simulink model "power_mosfet_device"  (R2025b)
settings: Solver=ode23tb  StartTime=0.0  StopTime=simlength  MaxStep=tc  RelTol=1e-3
values from neighbouring files (symbols this model uses):
  freq = 20e3    (= 20000)    [init_model.m]
  m = 0.5    [init_model.m]
  Rgate_turn_off = 1e-3    (= 0.001)    [init_model.m]
  Rgate_turn_on = 1    [init_model.m]
undefined symbols (not defined in the file or in its folder): cp_al, DThs_init, mosfet, Rth_mosfet_HA, Tambient, weigth
libraries: fl_lib x68, nesl_utility x32, simulink x4, advanced_mosfet_lib x2, basic_mosfet_lib x1, ee_lib x1
(part 1 of 2)
settings Model: SimulationMode=accelerator  Creator=dbagn  LastModifiedBy=dbagn

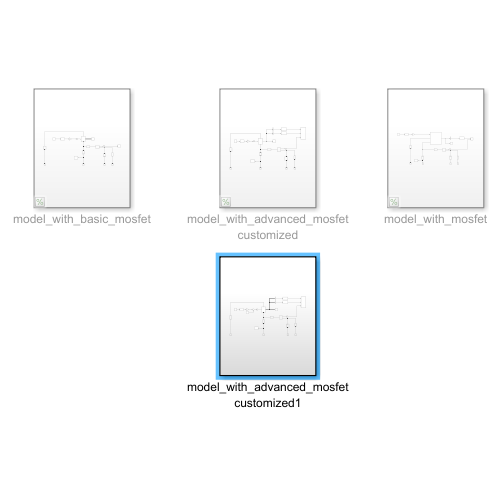
[thumbnail: Simulink's stored preview of the top-level diagram]
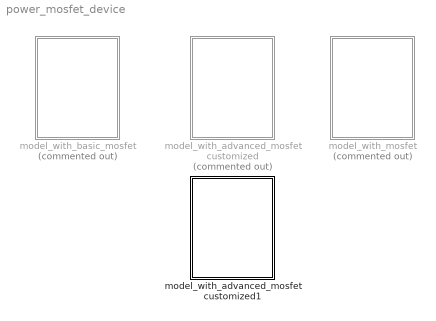
== system power_mosfet_device ==
  model_with_advanced_mosfet customized : Subsystem  Commented=on
  model_with_advanced_mosfet customized1 : Subsystem
  model_with_basic_mosfet : Subsystem  Commented=on
  model_with_mosfet : Subsystem  Commented=on

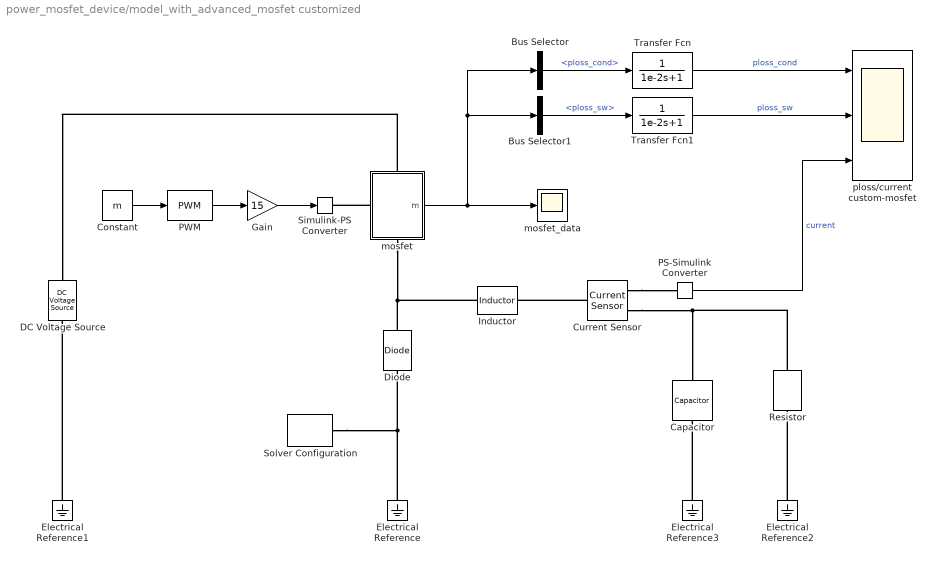
== system power_mosfet_device/model_with_advanced_mosfet customized ==
  Bus Selector : BusSelector  OutputSignals=basic_mosfet.ploss_cond
  Bus Selector1 : BusSelector  OutputSignals=basic_mosfet.ploss_sw
  Capacitor : fl_lib/Electrical/Electrical Elements/Capacitor  c=C F  r=1e-6 Ohm  g=0 1/Ohm  i_specify=off  i_priority=None  i=0 A  i_nominal_specify=off  i_nominal_value=1  i_nominal_unit=A  v_specify=off  v_priority=None  v=0 V  v_nominal_specify=off  v_nominal_value=1  v_nominal_unit=V  vc_specify=off  vc_priority=High  vc=0 V  vc_nominal_specify=off  vc_nominal_value=1  vc_nominal_unit=V
  Constant : Constant  Value=m
  Current Sensor : fl_lib/Electrical/Electrical Sensors/Current Sensor
  DC Voltage Source : fl_lib/Electrical/Electrical Sources/DC Voltage Source  v0=600 V
  Diode : fl_lib/Electrical/Electrical Elements/Diode  Vf=0.35 V  Ron=1e-3 Ohm  Goff=1e-8 1/Ohm  i_specify=off  i_priority=None  i=0 A  i_nominal_specify=off  i_nominal_value=1  i_nominal_unit=A  v_specify=off  v_priority=None  v=0 V  v_nominal_specify=off  v_nominal_value=1  v_nominal_unit=V
  Electrical Reference{,1..3} (4 alike) : fl_lib/Electrical/Electrical Elements/Electrical Reference
  Gain : Gain  Gain=15
  Inductor : fl_lib/Electrical/Electrical Elements/Inductor  l=L H  r=2e-3 Ohm  g=1e-9 1/Ohm  i_specify=off  i_priority=None  i=0 A  i_nominal_specify=off  i_nominal_value=1  i_nominal_unit=A  v_specify=off  v_priority=None  v=0 V  v_nominal_specify=off  v_nominal_value=1  v_nominal_unit=V  i_L_specify=off  i_L_priority=High  i_L=0 A  i_L_nominal_specify=off  i_L_nominal_value=1  i_L_nominal_unit=A
  PS-Simulink Converter : nesl_utility/PS-Simulink Converter  PhysicalDomain=network_engine_domain  SubClassName=ps_output  LeftPortType=input  RightPortType=output  PseudoPeriodic=off  Frequencies=[]  VectorFormat=1-D array  Unit=A  AffineConversion=off
  PWM : simulink/Discontinuities/PWM  DisableCoverage=on  Period=1/freq  InitialDelay=0  DisallowZeroDutyCycle=off  RunAtFixedTimeIntervals=off  SampleTime=0.1
  Resistor : fl_lib/Electrical/Electrical Elements/Resistor  R=300/200 Ohm  i_specify=off  i_priority=None  i=0 A  i_nominal_specify=off  i_nominal_value=1  i_nominal_unit=A  v_specify=off  v_priority=None  v=0 V  v_nominal_specify=off  v_nominal_value=1  v_nominal_unit=V
  Simulink-PS Converter : nesl_utility/Simulink-PS Converter  PhysicalDomain=network_engine_domain  SubClassName=ps_input  LeftPortType=input  RightPortType=output  PseudoPeriodic=off  Frequencies=[]  NoiseDistribution=none  NoiseParameters=[]  Unit=1  AffineConversion=off  FilteringAndDerivatives=provide  SimscapeFilterOrder=1  InputFilterTimeConstant=0.001  UdotUserProvided=0
  Solver Configuration : nesl_utility/Solver Configuration  PhysicalDomain=network_engine_domain  SubClassName=solver  LeftPortType=input  RightPortType=generic  Tones=[]  Harmonics=[]  SimulateNoise=off  Profile=off  UseLocalSampling=off  EnableSwitchedLinearOptims=on  FrequencyDomain=off  UseCCode=off  RelTol=0.001  AbsTol=0.001  MinStep=1e-09  ToWorkspace=off  RevertToSquareIcSolve=off  NumHomotopyIterations=100  PhasorMode=off  PhasorModeNumHarmonics=1  ConsistencySolver=NEWTON_XTOL_AFTER_FTOL  IndexReductionMethod=DerivativeReplacement  DoDC=on  ResidualTolerance=1e-09  ConsistencyTolSource=GLOBAL  ConsistencyAbsTol=0.001  ConsistencyRelTol=0.001  ConsistencyTolFactor=0.001  UseLocalSolver=on  LocalSolverChoice=NE_BACKWARD_EULER_ADVANCER  ResolveIndetEquations=on  FunctionEvalNumThread=1  LocalSolverSampleTime=tc  DoFixedCost=on  MaxNonlinIter=3  MaxModeIter=2  ComputeImpulses=off  ImpulseIterations=2  LinearAlgebra=auto  LinearAlgebraNumThread=0  EquationFormulation=NE_TIME_EF  DelaysMemoryBudget=1024  AutomaticFiltering=on  FilteringTimeConstant=0.001  PartitionStorageMethod=AS_NEEDED  PartitionMemoryBudget=1024  PartitionMethod=ROBUST  MultibodyUseLocalSolver=off  MultibodyLocalSolverChoice=ODE1  MultibodyLocalSolverSampleTime=0.001
  Transfer Fcn : TransferFcn  Denominator=[1e-2 1]
  Transfer Fcn1 : TransferFcn  Denominator=[1e-2 1]
  mosfet : Subsystem  mask{Rds_on_m=mosfet.inv.Rds_on, Vth_m=mosfet.inv.Vth, Vdon_diode_m=mosfet.inv.Vdon_diode, Rdon_diode_m=mosfet.inv.Rdon_diode, g_fs_m=mosfet.inv.g_fs, Cgs_m=mosfet.inv.Cgs, Cgd_m=mosfet.inv.Cgd, Cds_m=mosfet.inv.Cds, Eon_m=mosfet.inv.Eon, Eoff_m=mosfet.inv.Eoff, Err_m=mosfet.inv.Erec, Voff_sw_loss_m=mosfet.inv.Voff_sw_losses, Ion_sw_loss_m=mosfet.inv.Ion_sw_losses, Rgate_internal_m=mosfet.inv.Rgate_internal, Rgate_turn_on_m=Rgate_turn_on, Rgate_turn_off_m=Rgate_turn_off, Lstray_m=mosfet.inv.Lstray_module}
      mask prompts: Rds_on_m "Rds_on (Ohm)"; Vth_m "Vth (V)"; Vdon_diode_m "Vdon_diode (V)"; Rdon_diode_m "Rdon_diode (Ohm)"; g_fs_m "g_fs (A/V)"; Cgs_m "Cgs (F)"; Cgd_m "Cgd (F)"; Cds_m "Cds (F)"; Eon_m "Eon (J)"; Eoff_m "Eoff (J)"; Err_m "Err (J)"; Voff_sw_loss_m "Voff_sw_loss (V)"; Ion_sw_loss_m "Ion _sw_loss (A)"; Rgate_internal_m "Rgate internal (Ohm)"; Rgate_turn_on_m "Rgate turn on (Ohm)"; Rgate_turn_off_m "Rgate turn off (Ohm)"; Lstray_m "Lstray module (H)"
      settings: PortSchema="{\"entries\":[{\"content\":{\"sides\":[{\"content\":{\"connectorIds\":[\"LConn1\"]},\"type\":\"ConnectorPlacement.EquallySpacedRectSide\",\"uuid\":\"325dc963-858c-47f0-8995-f323ab4d9c46\"},{\"content\":{\"connectorIds\":[\"Out1\"],\"side\":\"RIGHT\"},\"type\":\"ConnectorPlacement.EquallySpacedRectSide\",\"uuid\":\"e9e66084-ecb2-40fb-9a1e-77677e0cc1df\"},{\"content\":{\"connectorIds\":[\"LConn2\"],\"side\":\"TOP\"},\"type\":\"ConnectorPlacement.EquallySpacedRectSide\",\"uuid\":\"9480d797-f2f6-459b-bb7c-d63861b57fde\"},{\"content\":{\"connectorIds\":[\"RConn1\"],\"side\":\"BOTTOM\"},\"type\":\"ConnectorPlacement.EquallySpacedRectSide\",\"uuid\":\"b13176d9-73b9-4822-9a0d-ec75065272bc\"}]},\"type\":\"ConnectorPlacement.EquallySpacedConnector\",\"uuid\":\"5e4a07d9-f5e8-4613-9049-5a866b5d2453\"}],\"packageUris\":[\"http://schema.mathworks.com/mf0/Connector/R2020b\"],\"version\":\"1.0\"}"
  mosfet_data : Scope
      settings: SampleTime=tc  ActiveDisplayYMinimum=-130.18028660470713  ActiveDisplayYMaximum=1171.6225788682864
  ploss/current custom-mosfet : Scope  NumInputPorts=3
      settings: ActiveDisplayYMinimum=-4.6879645806866894E+6  ActiveDisplayYMaximum=4.2191681226180211E+7
  wires:
  Gain/1 -> Simulink-PS Converter/1
  mosfet/1(m) -> Bus Selector1/1, Bus Selector/1, mosfet_data/1
  Constant/1 -> PWM/1
  PWM/1 -> Gain/1
  Bus Selector/1 -> Transfer Fcn/1  "<ploss_cond>"
  Transfer Fcn/1 -> ploss/current custom-mosfet/1  "ploss_cond"
  PS-Simulink Converter/1 -> ploss/current custom-mosfet/3  "current"
  Bus Selector1/1 -> Transfer Fcn1/1  "<ploss_sw>"
  Transfer Fcn1/1 -> ploss/current custom-mosfet/2  "ploss_sw"
  connections:
  Electrical Reference1/LConn1 -- DC Voltage Source/RConn1
  mosfet/LConn1 -- Simulink-PS Converter/RConn1
  mosfet/LConn2 -- Diode/RConn1 -- Inductor/LConn1
  Resistor/LConn1 -- Capacitor/LConn1 -- Current Sensor/RConn2
  Electrical Reference2/LConn1 -- Resistor/RConn1
  Electrical Reference3/LConn1 -- Capacitor/RConn1
  Solver Configuration/RConn1 -- Electrical Reference/LConn1 -- Diode/LConn1
  mosfet/RConn1 -- DC Voltage Source/LConn1
  Current Sensor/LConn1 -- Inductor/RConn1
  Current Sensor/RConn1 -- PS-Simulink Converter/LConn1

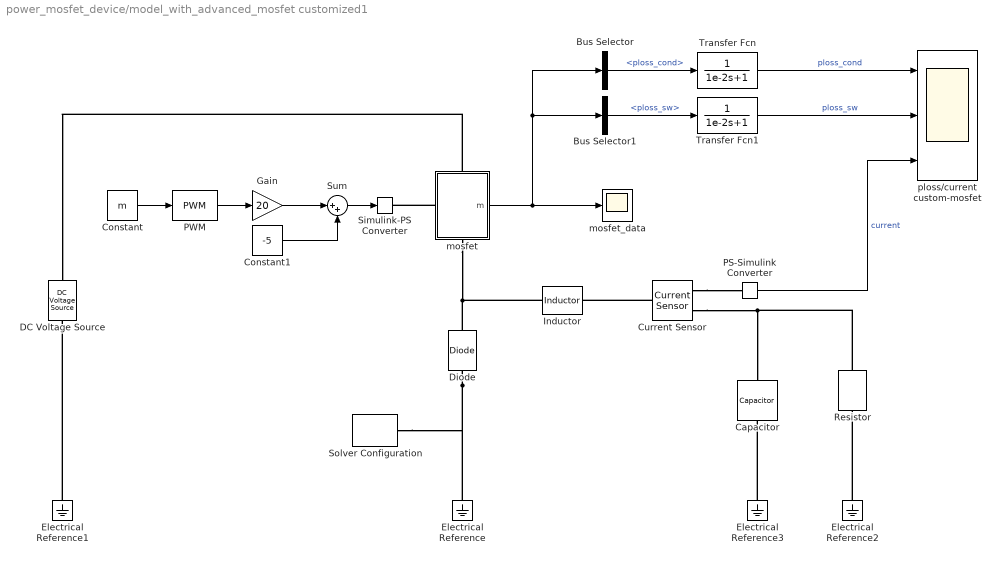
== system power_mosfet_device/model_with_advanced_mosfet customized1 ==
  Bus Selector : BusSelector  OutputSignals=basic_mosfet.ploss_cond
  Bus Selector1 : BusSelector  OutputSignals=basic_mosfet.ploss_sw
  Capacitor : fl_lib/Electrical/Electrical Elements/Capacitor  c=C F  r=1e-6 Ohm  g=0 1/Ohm  i_specify=off  i_priority=None  i=0 A  i_nominal_specify=off  i_nominal_value=1  i_nominal_unit=A  v_specify=off  v_priority=None  v=0 V  v_nominal_specify=off  v_nominal_value=1  v_nominal_unit=V  vc_specify=off  vc_priority=High  vc=0 V  vc_nominal_specify=off  vc_nominal_value=1  vc_nominal_unit=V
  Constant : Constant  Value=m
  Constant1 : Constant  Value=-5
  Current Sensor : fl_lib/Electrical/Electrical Sensors/Current Sensor
  DC Voltage Source : fl_lib/Electrical/Electrical Sources/DC Voltage Source  v0=600 V
  Diode : fl_lib/Electrical/Electrical Elements/Diode  Vf=0.35 V  Ron=1e-3 Ohm  Goff=1e-8 1/Ohm  i_specify=off  i_priority=None  i=0 A  i_nominal_specify=off  i_nominal_value=1  i_nominal_unit=A  v_specify=off  v_priority=None  v=0 V  v_nominal_specify=off  v_nominal_value=1  v_nominal_unit=V
  Electrical Reference{,1..3} (4 alike) : fl_lib/Electrical/Electrical Elements/Electrical Reference
  Gain : Gain  Gain=20
  Inductor : fl_lib/Electrical/Electrical Elements/Inductor  l=L H  r=2e-3 Ohm  g=1e-9 1/Ohm  i_specify=off  i_priority=None  i=0 A  i_nominal_specify=off  i_nominal_value=1  i_nominal_unit=A  v_specify=off  v_priority=None  v=0 V  v_nominal_specify=off  v_nominal_value=1  v_nominal_unit=V  i_L_specify=off  i_L_priority=High  i_L=0 A  i_L_nominal_specify=off  i_L_nominal_value=1  i_L_nominal_unit=A
  PS-Simulink Converter : nesl_utility/PS-Simulink Converter  PhysicalDomain=network_engine_domain  SubClassName=ps_output  LeftPortType=input  RightPortType=output  PseudoPeriodic=off  Frequencies=[]  VectorFormat=1-D array  Unit=A  AffineConversion=off
  PWM : simulink/Discontinuities/PWM  DisableCoverage=on  Period=1/freq  InitialDelay=0  DisallowZeroDutyCycle=off  RunAtFixedTimeIntervals=off  SampleTime=0.1
  Resistor : fl_lib/Electrical/Electrical Elements/Resistor  R=300/200 Ohm  i_specify=off  i_priority=None  i=0 A  i_nominal_specify=off  i_nominal_value=1  i_nominal_unit=A  v_specify=off  v_priority=None  v=0 V  v_nominal_specify=off  v_nominal_value=1  v_nominal_unit=V
  Simulink-PS Converter : nesl_utility/Simulink-PS Converter  PhysicalDomain=network_engine_domain  SubClassName=ps_input  LeftPortType=input  RightPortType=output  PseudoPeriodic=off  Frequencies=[]  NoiseDistribution=none  NoiseParameters=[]  Unit=1  AffineConversion=off  FilteringAndDerivatives=provide  SimscapeFilterOrder=1  InputFilterTimeConstant=0.001  UdotUserProvided=0
  Solver Configuration : nesl_utility/Solver Configuration  PhysicalDomain=network_engine_domain  SubClassName=solver  LeftPortType=input  RightPortType=generic  Tones=[]  Harmonics=[]  SimulateNoise=off  Profile=off  UseLocalSampling=off  EnableSwitchedLinearOptims=on  FrequencyDomain=off  UseCCode=off  RelTol=0.001  AbsTol=0.001  MinStep=1e-09  ToWorkspace=off  RevertToSquareIcSolve=off  NumHomotopyIterations=100  PhasorMode=off  PhasorModeNumHarmonics=1  ConsistencySolver=NEWTON_XTOL_AFTER_FTOL  IndexReductionMethod=DerivativeReplacement  DoDC=on  ResidualTolerance=1e-09  ConsistencyTolSource=GLOBAL  ConsistencyAbsTol=0.001  ConsistencyRelTol=0.001  ConsistencyTolFactor=0.001  UseLocalSolver=on  LocalSolverChoice=NE_BACKWARD_EULER_ADVANCER  ResolveIndetEquations=on  FunctionEvalNumThread=1  LocalSolverSampleTime=tc  DoFixedCost=on  MaxNonlinIter=3  MaxModeIter=2  ComputeImpulses=off  ImpulseIterations=2  LinearAlgebra=auto  LinearAlgebraNumThread=0  EquationFormulation=NE_TIME_EF  DelaysMemoryBudget=1024  AutomaticFiltering=on  FilteringTimeConstant=0.001  PartitionStorageMethod=AS_NEEDED  PartitionMemoryBudget=1024  PartitionMethod=ROBUST  MultibodyUseLocalSolver=off  MultibodyLocalSolverChoice=ODE1  MultibodyLocalSolverSampleTime=0.001
  Sum : Sum  Inputs=|++
  Transfer Fcn : TransferFcn  Denominator=[1e-2 1]
  Transfer Fcn1 : TransferFcn  Denominator=[1e-2 1]
  mosfet : Subsystem  mask{Rds_on_m=mosfet.inv.Rds_on, Vth_m=mosfet.inv.Vth, Vdon_diode_m=mosfet.inv.Vdon_diode, Rdon_diode_m=mosfet.inv.Rdon_diode, g_fs_m=mosfet.inv.g_fs, Cgs_m=mosfet.inv.Cgs, Cgd_m=mosfet.inv.Cgd, Cds_m=mosfet.inv.Cds, Eon_m=mosfet.inv.Eon, Eoff_m=mosfet.inv.Eoff, Err_m=mosfet.inv.Erec, Voff_sw_loss_m=mosfet.inv.Voff_sw_losses, Ion_sw_loss_m=mosfet.inv.Ion_sw_losses, Rgate_internal_m=mosfet.inv.Rgate_internal, Rgate_turn_on_m=Rgate_turn_on, Rgate_turn_off_m=Rgate_turn_off, Lstray_m=mosfet.inv.Lstray_module}
      mask prompts: Rds_on_m "Rds_on (Ohm)"; Vth_m "Vth (V)"; Vdon_diode_m "Vdon_diode (V)"; Rdon_diode_m "Rdon_diode (Ohm)"; g_fs_m "g_fs (A/V)"; Cgs_m "Cgs (F)"; Cgd_m "Cgd (F)"; Cds_m "Cds (F)"; Eon_m "Eon (J)"; Eoff_m "Eoff (J)"; Err_m "Err (J)"; Voff_sw_loss_m "Voff_sw_loss (V)"; Ion_sw_loss_m "Ion _sw_loss (A)"; Rgate_internal_m "Rgate internal (Ohm)"; Rgate_turn_on_m "Rgate turn on (Ohm)"; Rgate_turn_off_m "Rgate turn off (Ohm)"; Lstray_m "Lstray module (H)"
      settings: PortSchema="{\"entries\":[{\"content\":{\"sides\":[{\"content\":{\"connectorIds\":[\"LConn1\"]},\"type\":\"ConnectorPlacement.EquallySpacedRectSide\",\"uuid\":\"325dc963-858c-47f0-8995-f323ab4d9c46\"},{\"content\":{\"connectorIds\":[\"Out1\"],\"side\":\"RIGHT\"},\"type\":\"ConnectorPlacement.EquallySpacedRectSide\",\"uuid\":\"e9e66084-ecb2-40fb-9a1e-77677e0cc1df\"},{\"content\":{\"connectorIds\":[\"LConn2\"],\"side\":\"TOP\"},\"type\":\"ConnectorPlacement.EquallySpacedRectSide\",\"uuid\":\"9480d797-f2f6-459b-bb7c-d63861b57fde\"},{\"content\":{\"connectorIds\":[\"RConn1\"],\"side\":\"BOTTOM\"},\"type\":\"ConnectorPlacement.EquallySpacedRectSide\",\"uuid\":\"b13176d9-73b9-4822-9a0d-ec75065272bc\"}]},\"type\":\"ConnectorPlacement.EquallySpacedConnector\",\"uuid\":\"5e4a07d9-f5e8-4613-9049-5a866b5d2453\"}],\"packageUris\":[\"http://schema.mathworks.com/mf0/Connector/R2020b\"],\"version\":\"1.0\"}"
  mosfet_data : Scope
      settings: SampleTime=tc  ActiveDisplayYMinimum=-1205.322347971507  ActiveDisplayYMaximum=2898.4652473437918
  ploss/current custom-mosfet : Scope  NumInputPorts=3
      settings: ActiveDisplayYMinimum=-1.5081366929735125  ActiveDisplayYMaximum=13.573230236761617
  wires:
  Transfer Fcn1/1 -> ploss/current custom-mosfet/2  "ploss_sw"
  Bus Selector1/1 -> Transfer Fcn1/1  "<ploss_sw>"
  PS-Simulink Converter/1 -> ploss/current custom-mosfet/3  "current"
  Transfer Fcn/1 -> ploss/current custom-mosfet/1  "ploss_cond"
  Bus Selector/1 -> Transfer Fcn/1  "<ploss_cond>"
  PWM/1 -> Gain/1
  Constant/1 -> PWM/1
  mosfet/1(m) -> mosfet_data/1, Bus Selector/1, Bus Selector1/1
  Gain/1 -> Sum/1
  Sum/1 -> Simulink-PS Converter/1
  Constant1/1 -> Sum/2
  connections:
  Current Sensor/RConn1 -- PS-Simulink Converter/LConn1
  Current Sensor/LConn1 -- Inductor/RConn1
  mosfet/RConn1 -- DC Voltage Source/LConn1
  Diode/LConn1 -- Electrical Reference/LConn1 -- Solver Configuration/RConn1
  Electrical Reference3/LConn1 -- Capacitor/RConn1
  Electrical Reference2/LConn1 -- Resistor/RConn1
  Current Sensor/RConn2 -- Capacitor/LConn1 -- Resistor/LConn1
  Inductor/LConn1 -- Diode/RConn1 -- mosfet/LConn2
  mosfet/LConn1 -- Simulink-PS Converter/RConn1
  Electrical Reference1/LConn1 -- DC Voltage Source/RConn1

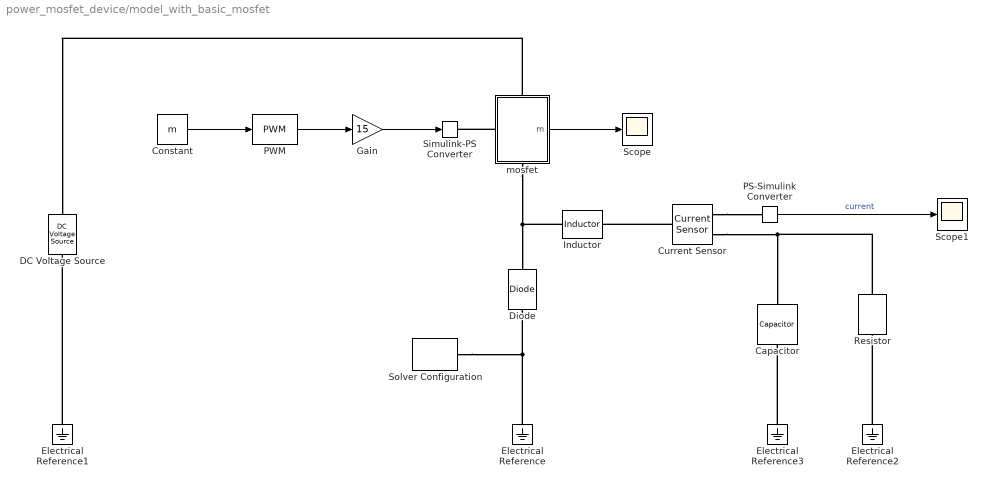
== system power_mosfet_device/model_with_basic_mosfet ==
  Capacitor : fl_lib/Electrical/Electrical Elements/Capacitor  c=C F  r=1e-6 Ohm  g=0 1/Ohm  i_specify=off  i_priority=None  i=0 A  i_nominal_specify=off  i_nominal_value=1  i_nominal_unit=A  v_specify=off  v_priority=None  v=0 V  v_nominal_specify=off  v_nominal_value=1  v_nominal_unit=V  vc_specify=off  vc_priority=High  vc=0 V  vc_nominal_specify=off  vc_nominal_value=1  vc_nominal_unit=V
  Constant : Constant  Value=m
  Current Sensor : fl_lib/Electrical/Electrical Sensors/Current Sensor
  DC Voltage Source : fl_lib/Electrical/Electrical Sources/DC Voltage Source  v0=600 V
  Diode : fl_lib/Electrical/Electrical Elements/Diode  Vf=0.35 V  Ron=1e-3 Ohm  Goff=1e-8 1/Ohm  i_specify=off  i_priority=None  i=0 A  i_nominal_specify=off  i_nominal_value=1  i_nominal_unit=A  v_specify=off  v_priority=None  v=0 V  v_nominal_specify=off  v_nominal_value=1  v_nominal_unit=V
  Electrical Reference{,1..3} (4 alike) : fl_lib/Electrical/Electrical Elements/Electrical Reference
  Gain : Gain  Gain=15
  Inductor : fl_lib/Electrical/Electrical Elements/Inductor  l=L H  r=2e-3 Ohm  g=1e-9 1/Ohm  i_specify=off  i_priority=None  i=0 A  i_nominal_specify=off  i_nominal_value=1  i_nominal_unit=A  v_specify=off  v_priority=None  v=0 V  v_nominal_specify=off  v_nominal_value=1  v_nominal_unit=V  i_L_specify=off  i_L_priority=High  i_L=0 A  i_L_nominal_specify=off  i_L_nominal_value=1  i_L_nominal_unit=A
  PS-Simulink Converter : nesl_utility/PS-Simulink Converter  PhysicalDomain=network_engine_domain  SubClassName=ps_output  LeftPortType=input  RightPortType=output  PseudoPeriodic=off  Frequencies=[]  VectorFormat=1-D array  Unit=A  AffineConversion=off
  PWM : simulink/Discontinuities/PWM  DisableCoverage=on  Period=1/freq  InitialDelay=0  DisallowZeroDutyCycle=off  RunAtFixedTimeIntervals=off  SampleTime=0.1
  Resistor : fl_lib/Electrical/Electrical Elements/Resistor  R=300/200 Ohm  i_specify=off  i_priority=None  i=0 A  i_nominal_specify=off  i_nominal_value=1  i_nominal_unit=A  v_specify=off  v_priority=None  v=0 V  v_nominal_specify=off  v_nominal_value=1  v_nominal_unit=V
  Scope : Scope
      settings: SampleTime=tc  ActiveDisplayYMinimum=-75.266839616145688  ActiveDisplayYMaximum=677.40155654531134
  Scope1 : Scope
      settings: SampleTime=tc  ActiveDisplayYMinimum=159.93430922640852  ActiveDisplayYMaximum=242.39946565162148  DataLoggingVariableName=ScopeData2
  Simulink-PS Converter : nesl_utility/Simulink-PS Converter  PhysicalDomain=network_engine_domain  SubClassName=ps_input  LeftPortType=input  RightPortType=output  PseudoPeriodic=off  Frequencies=[]  NoiseDistribution=none  NoiseParameters=[]  Unit=1  AffineConversion=off  FilteringAndDerivatives=provide  SimscapeFilterOrder=1  InputFilterTimeConstant=0.001  UdotUserProvided=0
  Solver Configuration : nesl_utility/Solver Configuration  PhysicalDomain=network_engine_domain  SubClassName=solver  LeftPortType=input  RightPortType=generic  Tones=[]  Harmonics=[]  SimulateNoise=off  Profile=off  UseLocalSampling=off  EnableSwitchedLinearOptims=on  FrequencyDomain=off  UseCCode=off  RelTol=0.001  AbsTol=0.001  MinStep=1e-09  ToWorkspace=off  RevertToSquareIcSolve=off  NumHomotopyIterations=100  PhasorMode=off  PhasorModeNumHarmonics=1  ConsistencySolver=NEWTON_XTOL_AFTER_FTOL  IndexReductionMethod=DerivativeReplacement  DoDC=on  ResidualTolerance=1e-09  ConsistencyTolSource=GLOBAL  ConsistencyAbsTol=0.001  ConsistencyRelTol=0.001  ConsistencyTolFactor=0.001  UseLocalSolver=on  LocalSolverChoice=NE_BACKWARD_EULER_ADVANCER  ResolveIndetEquations=on  FunctionEvalNumThread=1  LocalSolverSampleTime=tc  DoFixedCost=on  MaxNonlinIter=3  MaxModeIter=2  ComputeImpulses=off  ImpulseIterations=2  LinearAlgebra=auto  LinearAlgebraNumThread=0  EquationFormulation=NE_TIME_EF  DelaysMemoryBudget=1024  AutomaticFiltering=on  FilteringTimeConstant=0.001  PartitionStorageMethod=AS_NEEDED  PartitionMemoryBudget=1024  PartitionMethod=ROBUST  MultibodyUseLocalSolver=off  MultibodyLocalSolverChoice=ODE1  MultibodyLocalSolverSampleTime=0.001
  mosfet : Subsystem  mask{Rds_on=mosfet.inv.Rds_on, Vth=mosfet.inv.Vth, Csnubber=mosfet.inv.Csnubber, Rsnubber=mosfet.inv.Rsnubber, Lstray=mosfet.inv.Lstray_module/2, Vdon_diode=mosfet.inv.Vdon_diode, Rdon_diode=mosfet.inv.Rdon_diode, g_fs=mosfet.inv.g_fs}
      mask prompts: Rds_on "Rds_on (Ohm)"; Vth "Vth (V)"; Csnubber "Csnubber (F)"; Rsnubber "Rsnubber (Ohm)"; Lstray "Lstray (H)"; Vdon_diode "Vdon_diode (V)"; Rdon_diode "Rdon_diode (Ohm)"; g_fs "g_fs (A/V)"
      settings: PortSchema="{\"entries\":[{\"content\":{\"sides\":[{\"content\":{\"connectorIds\":[\"LConn1\"]},\"type\":\"ConnectorPlacement.EquallySpacedRectSide\",\"uuid\":\"325dc963-858c-47f0-8995-f323ab4d9c46\"},{\"content\":{\"connectorIds\":[\"Out1\"],\"side\":\"RIGHT\"},\"type\":\"ConnectorPlacement.EquallySpacedRectSide\",\"uuid\":\"e9e66084-ecb2-40fb-9a1e-77677e0cc1df\"},{\"content\":{\"connectorIds\":[\"LConn2\"],\"side\":\"TOP\"},\"type\":\"ConnectorPlacement.EquallySpacedRectSide\",\"uuid\":\"9480d797-f2f6-459b-bb7c-d63861b57fde\"},{\"content\":{\"connectorIds\":[\"RConn1\"],\"side\":\"BOTTOM\"},\"type\":\"ConnectorPlacement.EquallySpacedRectSide\",\"uuid\":\"b13176d9-73b9-4822-9a0d-ec75065272bc\"}]},\"type\":\"ConnectorPlacement.EquallySpacedConnector\",\"uuid\":\"5e4a07d9-f5e8-4613-9049-5a866b5d2453\"}],\"packageUris\":[\"http://schema.mathworks.com/mf0/Connector/R2020b\"],\"version\":\"1.0\"}"
  wires:
  PWM/1 -> Gain/1
  Constant/1 -> PWM/1
  mosfet/1(m) -> Scope/1
  Gain/1 -> Simulink-PS Converter/1
  PS-Simulink Converter/1 -> Scope1/1  "current"
  connections:
  mosfet/RConn1 -- DC Voltage Source/LConn1
  Electrical Reference/LConn1 -- Solver Configuration/RConn1 -- Diode/LConn1
  mosfet/LConn2 -- Inductor/LConn1 -- Diode/RConn1
  mosfet/LConn1 -- Simulink-PS Converter/RConn1
  Electrical Reference1/LConn1 -- DC Voltage Source/RConn1
  Current Sensor/RConn2 -- Resistor/LConn1 -- Capacitor/LConn1
  Current Sensor/LConn1 -- Inductor/RConn1
  Current Sensor/RConn1 -- PS-Simulink Converter/LConn1
  Electrical Reference2/LConn1 -- Resistor/RConn1
  Electrical Reference3/LConn1 -- Capacitor/RConn1

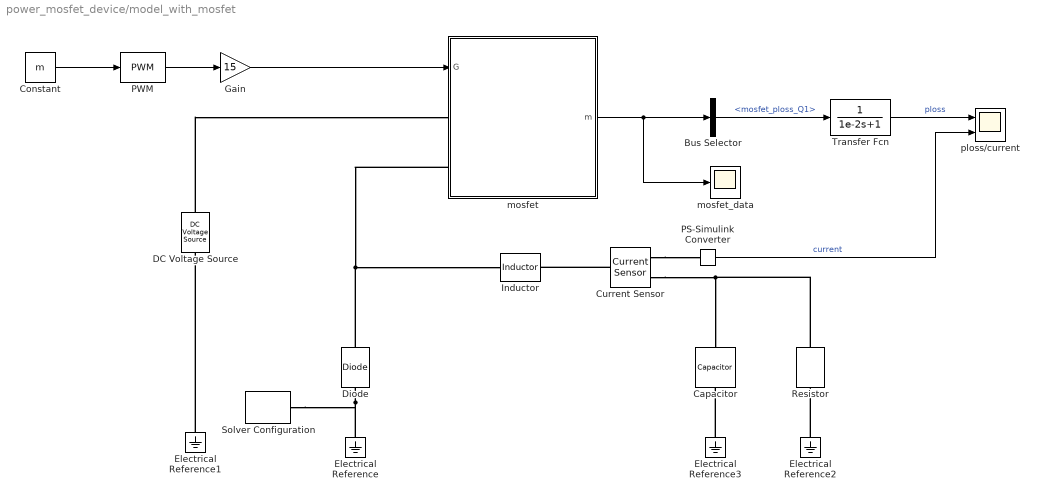
== system power_mosfet_device/model_with_mosfet ==
  Bus Selector : BusSelector  OutputSignals=mosfet_ploss_Q1
  Capacitor : fl_lib/Electrical/Electrical Elements/Capacitor  c=C F  r=1e-6 Ohm  g=0 1/Ohm  i_specify=off  i_priority=None  i=0 A  i_nominal_specify=off  i_nominal_value=1  i_nominal_unit=A  v_specify=off  v_priority=None  v=0 V  v_nominal_specify=off  v_nominal_value=1  v_nominal_unit=V  vc_specify=off  vc_priority=High  vc=0 V  vc_nominal_specify=off  vc_nominal_value=1  vc_nominal_unit=V
  Constant : Constant  Value=m
  Current Sensor : fl_lib/Electrical/Electrical Sensors/Current Sensor
  DC Voltage Source : fl_lib/Electrical/Electrical Sources/DC Voltage Source  v0=600 V
  Diode : fl_lib/Electrical/Electrical Elements/Diode  Vf=0.35 V  Ron=1e-3 Ohm  Goff=1e-8 1/Ohm  i_specify=off  i_priority=None  i=0 A  i_nominal_specify=off  i_nominal_value=1  i_nominal_unit=A  v_specify=off  v_priority=None  v=0 V  v_nominal_specify=off  v_nominal_value=1  v_nominal_unit=V
  Electrical Reference{,1..3} (4 alike) : fl_lib/Electrical/Electrical Elements/Electrical Reference
  Gain : Gain  Gain=15
  Inductor : fl_lib/Electrical/Electrical Elements/Inductor  l=L H  r=2e-3 Ohm  g=1e-9 1/Ohm  i_specify=off  i_priority=None  i=0 A  i_nominal_specify=off  i_nominal_value=1  i_nominal_unit=A  v_specify=off  v_priority=None  v=0 V  v_nominal_specify=off  v_nominal_value=1  v_nominal_unit=V  i_L_specify=off  i_L_priority=High  i_L=0 A  i_L_nominal_specify=off  i_L_nominal_value=1  i_L_nominal_unit=A
  PS-Simulink Converter : nesl_utility/PS-Simulink Converter  PhysicalDomain=network_engine_domain  SubClassName=ps_output  LeftPortType=input  RightPortType=output  PseudoPeriodic=off  Frequencies=[]  VectorFormat=1-D array  Unit=A  AffineConversion=off
  PWM : simulink/Discontinuities/PWM  DisableCoverage=on  Period=1/freq  InitialDelay=0  DisallowZeroDutyCycle=off  RunAtFixedTimeIntervals=off  SampleTime=0.1
  Resistor : fl_lib/Electrical/Electrical Elements/Resistor  R=300/200 Ohm  i_specify=off  i_priority=None  i=0 A  i_nominal_specify=off  i_nominal_value=1  i_nominal_unit=A  v_specify=off  v_priority=None  v=0 V  v_nominal_specify=off  v_nominal_value=1  v_nominal_unit=V
  Solver Configuration : nesl_utility/Solver Configuration  PhysicalDomain=network_engine_domain  SubClassName=solver  LeftPortType=input  RightPortType=generic  Tones=[]  Harmonics=[]  SimulateNoise=off  Profile=off  UseLocalSampling=off  EnableSwitchedLinearOptims=on  FrequencyDomain=off  UseCCode=off  RelTol=0.001  AbsTol=0.001  MinStep=1e-09  ToWorkspace=off  RevertToSquareIcSolve=off  NumHomotopyIterations=100  PhasorMode=off  PhasorModeNumHarmonics=1  ConsistencySolver=NEWTON_XTOL_AFTER_FTOL  IndexReductionMethod=DerivativeReplacement  DoDC=on  ResidualTolerance=1e-09  ConsistencyTolSource=GLOBAL  ConsistencyAbsTol=0.001  ConsistencyRelTol=0.001  ConsistencyTolFactor=0.001  UseLocalSolver=on  LocalSolverChoice=NE_BACKWARD_EULER_ADVANCER  ResolveIndetEquations=on  FunctionEvalNumThread=1  LocalSolverSampleTime=tc  DoFixedCost=on  MaxNonlinIter=3  MaxModeIter=2  ComputeImpulses=off  ImpulseIterations=2  LinearAlgebra=auto  LinearAlgebraNumThread=0  EquationFormulation=NE_TIME_EF  DelaysMemoryBudget=1024  AutomaticFiltering=on  FilteringTimeConstant=0.001  PartitionStorageMethod=AS_NEEDED  PartitionMemoryBudget=1024  PartitionMethod=ROBUST  MultibodyUseLocalSolver=off  MultibodyLocalSolverChoice=ODE1  MultibodyLocalSolverSampleTime=0.001
  Transfer Fcn : TransferFcn  Denominator=[1e-2 1]
  mosfet : Subsystem  mask{mass_heatsink=weigth, specific_heat=cp_al, rth_mosfet_HA=Rth_mosfet_HA, rth_mosfet_JH=mosfet.inv.Rth_switch_JH, Rds_on=mosfet.inv.Rds_on, Vth=mosfet.inv.Vth, Eon=mosfet.inv.Eon, Eoff=mosfet.inv.Eoff, Voff_sw_loss=mosfet.inv.Voff_sw_losses, Ion_sw_loss=mosfet.inv.Ion_sw_losses, Vdon_diode=mosfet.inv.Vdon_diode, Rdon_diode=mosfet.inv.Rdon_diode, JunctionTermalMass=mosfet.inv.JunctionTermalMass, Tambient=Tambient, DThs_init=DThs_init, Csnubber=mosfet.inv.Csnubber, Rsnubber=mosfet.inv.Rsnubber}
      mask prompts: mass_heatsink "Mass Heatsink (kg)"; specific_heat "Specific Heat (J/K/kg)"; rth_mosfet_HA "Thermal Resistance HA (K/W)"; rth_mosfet_JH "Thermal Resistance JH (K/W)"; Rds_on "Rds_on (Ohm)"; Vth "Vth (V)"; Eon "Eon (J)"; Eoff "Eoff (J)"; Voff_sw_loss "Voff_sw_loss (V)"; Ion_sw_loss "Ion_sw_loss (A)"; Vdon_diode "Vdon_diode (V)"; Rdon_diode "Rdon_diode (Ohm)"; JunctionTermalMass "JunctionTermalMass (J/K)"; Tambient "Tambient (degC)"; DThs_init "DThs_init (degC)"; Csnubber "Csnubber (F)"; Rsnubber "Rsnubber (Ohm)"
  mosfet_data : Scope
      settings: SampleTime=tc  ActiveDisplayYMinimum=-162.71512014835841  ActiveDisplayYMaximum=162.83727252978858
  ploss/current : Scope  NumInputPorts=2
      settings: ActiveDisplayYMinimum=112.87858768707648  ActiveDisplayYMaximum=429.36143412410507
  wires:
  PS-Simulink Converter/1 -> ploss/current/2  "current"
  Transfer Fcn/1 -> ploss/current/1  "ploss"
  Bus Selector/1 -> Transfer Fcn/1  "<mosfet_ploss_Q1>"
  PWM/1 -> Gain/1
  Constant/1 -> PWM/1
  Gain/1 -> mosfet/1(G)
  mosfet/1(m) -> mosfet_data/1, Bus Selector/1
  connections:
  Current Sensor/RConn1 -- PS-Simulink Converter/LConn1
  Current Sensor/LConn1 -- Inductor/RConn1
  Diode/LConn1 -- Electrical Reference/LConn1 -- Solver Configuration/RConn1
  Electrical Reference3/LConn1 -- Capacitor/RConn1
  Electrical Reference2/LConn1 -- Resistor/RConn1
  Current Sensor/RConn2 -- Capacitor/LConn1 -- Resistor/LConn1
  Diode/RConn1 -- mosfet/LConn2 -- Inductor/LConn1
  Electrical Reference1/LConn1 -- DC Voltage Source/RConn1
  DC Voltage Source/LConn1 -- mosfet/LConn1

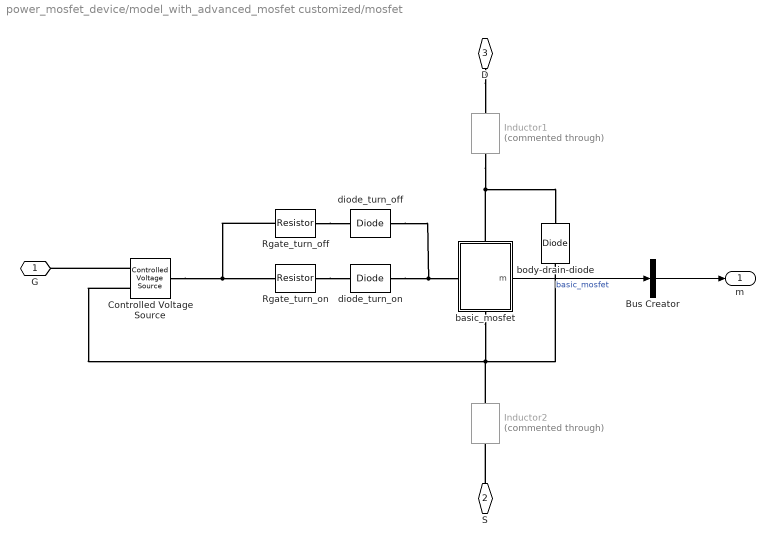
== system power_mosfet_device/model_with_advanced_mosfet customized/mosfet ==
  Bus Creator : BusCreator  Inputs=1
  Controlled Voltage Source : fl_lib/Electrical/Electrical Sources/Controlled Voltage Source
  Inductor1 : fl_lib/Electrical/Electrical Elements/Inductor  Commented=through  l=Lstray_m/2 H  r=0 Ohm  g=1e-9 1/Ohm  i_specify=off  i_priority=None  i=0 A  i_nominal_specify=off  i_nominal_value=1  i_nominal_unit=A  v_specify=off  v_priority=None  v=0 V  v_nominal_specify=off  v_nominal_value=1  v_nominal_unit=V  i_L_specify=off  i_L_priority=High  i_L=0 A  i_L_nominal_specify=off  i_L_nominal_value=1  i_L_nominal_unit=A
  Inductor2 : fl_lib/Electrical/Electrical Elements/Inductor  Commented=through  l=Lstray_m/2 H  r=0 Ohm  g=1e-9 1/Ohm  i_specify=off  i_priority=None  i=0 A  i_nominal_specify=off  i_nominal_value=1  i_nominal_unit=A  v_specify=off  v_priority=None  v=0 V  v_nominal_specify=off  v_nominal_value=1  v_nominal_unit=V  i_L_specify=off  i_L_priority=High  i_L=0 A  i_L_nominal_specify=off  i_L_nominal_value=1  i_L_nominal_unit=A
  Rgate_turn_off : fl_lib/Electrical/Electrical Elements/Resistor  R=Rgate_turn_off_m Ohm  i_specify=off  i_priority=None  i=0 A  i_nominal_specify=off  i_nominal_value=1  i_nominal_unit=A  v_specify=off  v_priority=None  v=0 V  v_nominal_specify=off  v_nominal_value=1  v_nominal_unit=V
  Rgate_turn_on : fl_lib/Electrical/Electrical Elements/Resistor  R=Rgate_turn_on_m Ohm  i_specify=off  i_priority=None  i=0 A  i_nominal_specify=off  i_nominal_value=1  i_nominal_unit=A  v_specify=off  v_priority=None  v=0 V  v_nominal_specify=off  v_nominal_value=1  v_nominal_unit=V
  basic_mosfet : Subsystem  mask{Vth_m=Vth_m, Rds_on_m=Rds_on_m, g_fs_m=g_fs_m, Cgs_m=Cgs_m, Cgd_m=Cgd_m, Cds_m=Cds_m, Eon_m=Eon_m, Eoff_m=Eoff_m, Err_m=Err_m, Voff_sw_loss_m=Voff_sw_loss_m, Ion_sw_loss_m=Ion_sw_loss_m, Rgate_internal=Rgate_internal_m}
      mask prompts: Vth_m "Vth (V)"; Rds_on_m "Rds_on (Ohm)"; g_fs_m "g_fs (A/V)"; Cgs_m "Cgs (F)"; Cgd_m "Cgd (F)"; Cds_m "Cds (F)"; Eon_m "Eon (J)"; Eoff_m "Eoff (J)"; Err_m "Err (J)"; Voff_sw_loss_m "Voff_sw_loss (V)"; Ion_sw_loss_m "Ion_sw_loss (A)"; Rgate_internal "Rgate internal (Ohm)"
      settings: PortSchema="{\"entries\":[{\"content\":{\"sides\":[{\"content\":{\"connectorIds\":[\"LConn1\"]},\"type\":\"ConnectorPlacement.EquallySpacedRectSide\",\"uuid\":\"325dc963-858c-47f0-8995-f323ab4d9c46\"},{\"content\":{\"connectorIds\":[\"Out1\"],\"side\":\"RIGHT\"},\"type\":\"ConnectorPlacement.EquallySpacedRectSide\",\"uuid\":\"e9e66084-ecb2-40fb-9a1e-77677e0cc1df\"},{\"content\":{\"connectorIds\":[\"LConn2\"],\"side\":\"TOP\"},\"type\":\"ConnectorPlacement.EquallySpacedRectSide\",\"uuid\":\"9480d797-f2f6-459b-bb7c-d63861b57fde\"},{\"content\":{\"connectorIds\":[\"RConn1\"],\"side\":\"BOTTOM\"},\"type\":\"ConnectorPlacement.EquallySpacedRectSide\",\"uuid\":\"bd6f7c3f-e73f-43a3-8bfd-bc4aa1f2c71d\"}]},\"type\":\"ConnectorPlacement.EquallySpacedConnector\",\"uuid\":\"5e4a07d9-f5e8-4613-9049-5a866b5d2453\"}],\"packageUris\":[\"http://schema.mathworks.com/mf0/Connector/R2020b\"],\"version\":\"1.0\"}"
  body-drain-diode : fl_lib/Electrical/Electrical Elements/Diode  Vf=Vdon_diode_m V  Ron=Rdon_diode_m Ohm  Goff=1e-8 1/Ohm  i_specify=off  i_priority=None  i=0 A  i_nominal_specify=off  i_nominal_value=1  i_nominal_unit=A  v_specify=off  v_priority=None  v=0 V  v_nominal_specify=off  v_nominal_value=1  v_nominal_unit=V
  diode_turn_off : fl_lib/Electrical/Electrical Elements/Diode  Vf=0.35 V  Ron=Rdon_diode_m Ohm  Goff=1e-8 1/Ohm  i_specify=off  i_priority=None  i=0 A  i_nominal_specify=off  i_nominal_value=1  i_nominal_unit=A  v_specify=off  v_priority=None  v=0 V  v_nominal_specify=off  v_nominal_value=1  v_nominal_unit=V
  diode_turn_on : fl_lib/Electrical/Electrical Elements/Diode  Vf=0.35 V  Ron=Rdon_diode_m Ohm  Goff=1e-8 1/Ohm  i_specify=off  i_priority=None  i=0 A  i_nominal_specify=off  i_nominal_value=1  i_nominal_unit=A  v_specify=off  v_priority=None  v=0 V  v_nominal_specify=off  v_nominal_value=1  v_nominal_unit=V
  G : PMIOPort  Side=Left
  S : PMIOPort  Port=2  Side=Left
  D : PMIOPort  Port=3  Side=Right
  m : Outport
  wires:
  basic_mosfet/1(m) -> Bus Creator/1  "basic_mosfet"
  Bus Creator/1 -> m/1
  connections:
  basic_mosfet/LConn2 -- Inductor1/LConn1 -- body-drain-diode/RConn1
  Controlled Voltage Source/RConn1 -- G/RConn1
  Controlled Voltage Source/LConn1 -- Rgate_turn_off/LConn1 -- Rgate_turn_on/LConn1
  Controlled Voltage Source/RConn2 -- Inductor2/RConn1 -- body-drain-diode/LConn1 -- basic_mosfet/RConn1
  D/RConn1 -- Inductor1/RConn1
  S/RConn1 -- Inductor2/LConn1
  Rgate_turn_on/RConn1 -- diode_turn_on/LConn1
  diode_turn_on/RConn1 -- diode_turn_off/LConn1 -- basic_mosfet/LConn1
  Rgate_turn_off/RConn1 -- diode_turn_off/RConn1

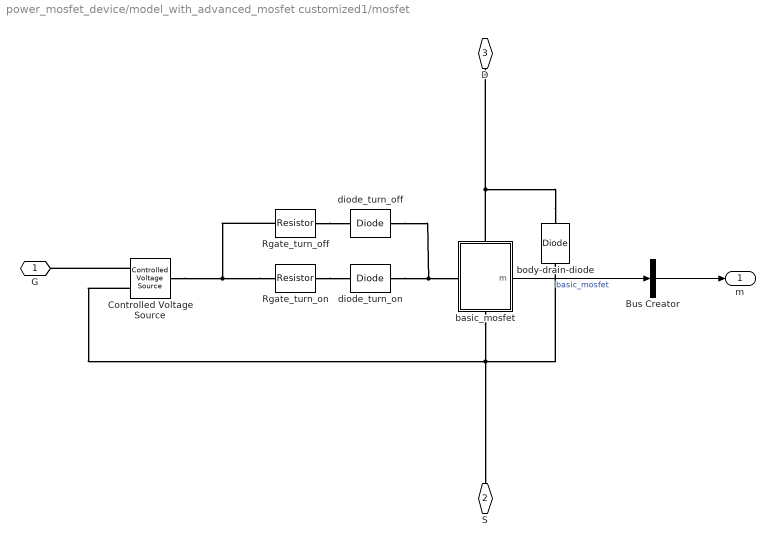
== system power_mosfet_device/model_with_advanced_mosfet customized1/mosfet ==
  Bus Creator : BusCreator  Inputs=1
  Controlled Voltage Source : fl_lib/Electrical/Electrical Sources/Controlled Voltage Source
  Rgate_turn_off : fl_lib/Electrical/Electrical Elements/Resistor  R=Rgate_turn_off_m Ohm  i_specify=off  i_priority=None  i=0 A  i_nominal_specify=off  i_nominal_value=1  i_nominal_unit=A  v_specify=off  v_priority=None  v=0 V  v_nominal_specify=off  v_nominal_value=1  v_nominal_unit=V
  Rgate_turn_on : fl_lib/Electrical/Electrical Elements/Resistor  R=Rgate_turn_on_m Ohm  i_specify=off  i_priority=None  i=0 A  i_nominal_specify=off  i_nominal_value=1  i_nominal_unit=A  v_specify=off  v_priority=None  v=0 V  v_nominal_specify=off  v_nominal_value=1  v_nominal_unit=V
  basic_mosfet : Subsystem  mask{Vth_m=Vth_m, Rds_on_m=Rds_on_m, g_fs_m=g_fs_m, Cgs_m=Cgs_m, Cgd_m=Cgd_m, Cds_m=Cds_m, Eon_m=Eon_m, Eoff_m=Eoff_m, Err_m=Err_m, Voff_sw_loss_m=Voff_sw_loss_m, Ion_sw_loss_m=Ion_sw_loss_m, Rgate_internal=Rgate_internal_m}
      mask prompts: Vth_m "Vth (V)"; Rds_on_m "Rds_on (Ohm)"; g_fs_m "g_fs (A/V)"; Cgs_m "Cgs (F)"; Cgd_m "Cgd (F)"; Cds_m "Cds (F)"; Eon_m "Eon (J)"; Eoff_m "Eoff (J)"; Err_m "Err (J)"; Voff_sw_loss_m "Voff_sw_loss (V)"; Ion_sw_loss_m "Ion_sw_loss (A)"; Rgate_internal "Rgate internal (Ohm)"
      settings: PortSchema="{\"entries\":[{\"content\":{\"sides\":[{\"content\":{\"connectorIds\":[\"LConn1\"]},\"type\":\"ConnectorPlacement.EquallySpacedRectSide\",\"uuid\":\"325dc963-858c-47f0-8995-f323ab4d9c46\"},{\"content\":{\"connectorIds\":[\"Out1\"],\"side\":\"RIGHT\"},\"type\":\"ConnectorPlacement.EquallySpacedRectSide\",\"uuid\":\"e9e66084-ecb2-40fb-9a1e-77677e0cc1df\"},{\"content\":{\"connectorIds\":[\"LConn2\"],\"side\":\"TOP\"},\"type\":\"ConnectorPlacement.EquallySpacedRectSide\",\"uuid\":\"9480d797-f2f6-459b-bb7c-d63861b57fde\"},{\"content\":{\"connectorIds\":[\"RConn1\"],\"side\":\"BOTTOM\"},\"type\":\"ConnectorPlacement.EquallySpacedRectSide\",\"uuid\":\"bd6f7c3f-e73f-43a3-8bfd-bc4aa1f2c71d\"}]},\"type\":\"ConnectorPlacement.EquallySpacedConnector\",\"uuid\":\"5e4a07d9-f5e8-4613-9049-5a866b5d2453\"}],\"packageUris\":[\"http://schema.mathworks.com/mf0/Connector/R2020b\"],\"version\":\"1.0\"}"
  body-drain-diode : fl_lib/Electrical/Electrical Elements/Diode  Vf=Vdon_diode_m V  Ron=Rdon_diode_m Ohm  Goff=1e-8 1/Ohm  i_specify=off  i_priority=None  i=0 A  i_nominal_specify=off  i_nominal_value=1  i_nominal_unit=A  v_specify=off  v_priority=None  v=0 V  v_nominal_specify=off  v_nominal_value=1  v_nominal_unit=V
  diode_turn_off : fl_lib/Electrical/Electrical Elements/Diode  Vf=0.35 V  Ron=Rdon_diode_m Ohm  Goff=1e-8 1/Ohm  i_specify=off  i_priority=None  i=0 A  i_nominal_specify=off  i_nominal_value=1  i_nominal_unit=A  v_specify=off  v_priority=None  v=0 V  v_nominal_specify=off  v_nominal_value=1  v_nominal_unit=V
  diode_turn_on : fl_lib/Electrical/Electrical Elements/Diode  Vf=0.35 V  Ron=Rdon_diode_m Ohm  Goff=1e-8 1/Ohm  i_specify=off  i_priority=None  i=0 A  i_nominal_specify=off  i_nominal_value=1  i_nominal_unit=A  v_specify=off  v_priority=None  v=0 V  v_nominal_specify=off  v_nominal_value=1  v_nominal_unit=V
  G : PMIOPort  Side=Left
  S : PMIOPort  Port=2  Side=Left
  D : PMIOPort  Port=3  Side=Right
  m : Outport
  wires:
  Bus Creator/1 -> m/1
  basic_mosfet/1(m) -> Bus Creator/1  "basic_mosfet"
  connections:
  Rgate_turn_off/RConn1 -- diode_turn_off/RConn1
  Rgate_turn_on/RConn1 -- diode_turn_on/LConn1
  basic_mosfet/RConn1 -- S/RConn1 -- body-drain-diode/LConn1 -- Controlled Voltage Source/RConn2
  body-drain-diode/RConn1 -- D/RConn1 -- basic_mosfet/LConn2
  Controlled Voltage Source/RConn1 -- G/RConn1
  Rgate_turn_on/LConn1 -- Rgate_turn_off/LConn1 -- Controlled Voltage Source/LConn1
  diode_turn_on/RConn1 -- basic_mosfet/LConn1 -- diode_turn_off/LConn1

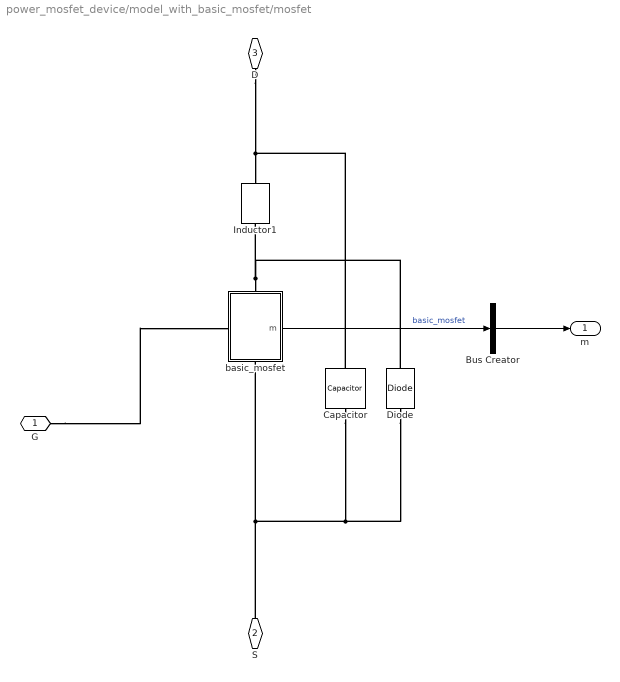
== system power_mosfet_device/model_with_basic_mosfet/mosfet ==
  Bus Creator : BusCreator  Inputs=1
  Capacitor : fl_lib/Electrical/Electrical Elements/Capacitor  c=Csnubber F  r=Rsnubber Ohm  g=0 1/Ohm  i_specify=off  i_priority=None  i=0 A  i_nominal_specify=off  i_nominal_value=1  i_nominal_unit=A  v_specify=off  v_priority=None  v=0 V  v_nominal_specify=off  v_nominal_value=1  v_nominal_unit=V  vc_specify=off  vc_priority=High  vc=0 V  vc_nominal_specify=off  vc_nominal_value=1  vc_nominal_unit=V
  Diode : fl_lib/Electrical/Electrical Elements/Diode  Vf=Vdon_diode V  Ron=Rdon_diode Ohm  Goff=1e-8 1/Ohm  i_specify=off  i_priority=None  i=0 A  i_nominal_specify=off  i_nominal_value=1  i_nominal_unit=A  v_specify=off  v_priority=None  v=0 V  v_nominal_specify=off  v_nominal_value=1  v_nominal_unit=V
  Inductor1 : fl_lib/Electrical/Electrical Elements/Inductor  l=Lstray H  r=0 Ohm  g=1e-9 1/Ohm  i_specify=off  i_priority=None  i=0 A  i_nominal_specify=off  i_nominal_value=1  i_nominal_unit=A  v_specify=off  v_priority=None  v=0 V  v_nominal_specify=off  v_nominal_value=1  v_nominal_unit=V  i_L_specify=off  i_L_priority=High  i_L=0 A  i_L_nominal_specify=off  i_L_nominal_value=1  i_L_nominal_unit=A
  basic_mosfet : Subsystem  mask{Vth=Vth, Rds_on=Rds_on, g_fs=g_fs}
      mask prompts: Vth "Vth (V)"; Rds_on "Rds_on (Ohm)"; g_fs "g_fs (A/V)"
      settings: PortSchema="{\"entries\":[{\"content\":{\"sides\":[{\"content\":{\"connectorIds\":[\"LConn1\"]},\"type\":\"ConnectorPlacement.EquallySpacedRectSide\",\"uuid\":\"325dc963-858c-47f0-8995-f323ab4d9c46\"},{\"content\":{\"connectorIds\":[\"Out1\"],\"side\":\"RIGHT\"},\"type\":\"ConnectorPlacement.EquallySpacedRectSide\",\"uuid\":\"e9e66084-ecb2-40fb-9a1e-77677e0cc1df\"},{\"content\":{\"connectorIds\":[\"LConn2\"],\"side\":\"TOP\"},\"type\":\"ConnectorPlacement.EquallySpacedRectSide\",\"uuid\":\"9480d797-f2f6-459b-bb7c-d63861b57fde\"},{\"content\":{\"connectorIds\":[\"RConn1\"],\"side\":\"BOTTOM\"},\"type\":\"ConnectorPlacement.EquallySpacedRectSide\",\"uuid\":\"bd6f7c3f-e73f-43a3-8bfd-bc4aa1f2c71d\"}]},\"type\":\"ConnectorPlacement.EquallySpacedConnector\",\"uuid\":\"5e4a07d9-f5e8-4613-9049-5a866b5d2453\"}],\"packageUris\":[\"http://schema.mathworks.com/mf0/Connector/R2020b\"],\"version\":\"1.0\"}"
  G : PMIOPort  Side=Left
  S : PMIOPort  Port=2  Side=Left
  D : PMIOPort  Port=3  Side=Right
  m : Outport
  wires:
  Bus Creator/1 -> m/1
  basic_mosfet/1(m) -> Bus Creator/1  "basic_mosfet"
  connections:
  Diode/LConn1 -- basic_mosfet/RConn1 -- S/RConn1 -- Capacitor/RConn1
  basic_mosfet/LConn2 -- Inductor1/LConn1 -- Diode/RConn1
  G/RConn1 -- basic_mosfet/LConn1
  Capacitor/LConn1 -- D/RConn1 -- Inductor1/RConn1

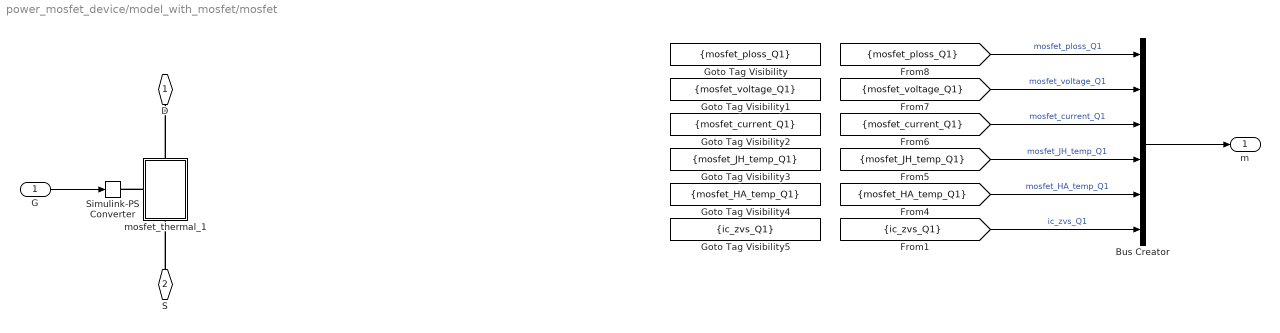
== system power_mosfet_device/model_with_mosfet/mosfet ==
  G : Inport
  Bus Creator : BusCreator  Inputs=6
  Goto Tag Visibility : GotoTagVisibility  GotoTag=mosfet_ploss_Q1
  Goto Tag Visibility1 : GotoTagVisibility  GotoTag=mosfet_voltage_Q1
  Goto Tag Visibility2 : GotoTagVisibility  GotoTag=mosfet_current_Q1
  Goto Tag Visibility3 : GotoTagVisibility  GotoTag=mosfet_JH_temp_Q1
  Goto Tag Visibility4 : GotoTagVisibility  GotoTag=mosfet_HA_temp_Q1
  Goto Tag Visibility5 : GotoTagVisibility  GotoTag=ic_zvs_Q1
  Simulink-PS Converter : nesl_utility/Simulink-PS Converter  PhysicalDomain=network_engine_domain  SubClassName=ps_input  LeftPortType=input  RightPortType=output  PseudoPeriodic=off  Frequencies=[]  NoiseDistribution=none  NoiseParameters=[]  Unit=V  AffineConversion=off  FilteringAndDerivatives=provide  SimscapeFilterOrder=1  InputFilterTimeConstant=0.001  UdotUserProvided=0
  mosfet_thermal_1 : Subsystem
      settings: PortSchema="{\"entries\":[{\"content\":{\"sides\":[{\"content\":{\"connectorIds\":[\"LConn1\"]},\"type\":\"ConnectorPlacement.EquallySpacedRectSide\",\"uuid\":\"9277da8d-d460-43e6-8478-dd662f15d226\"},{\"content\":{\"connectorIds\":[],\"side\":\"RIGHT\"},\"type\":\"ConnectorPlacement.EquallySpacedRectSide\",\"uuid\":\"a7ece396-f1d9-4f4f-a05b-db1fc65d6e1d\"},{\"content\":{\"connectorIds\":[\"LConn2\"],\"side\":\"TOP\"},\"type\":\"ConnectorPlacement.EquallySpacedRectSide\",\"uuid\":\"fdd70777-e9cf-4317-afb6-cae87f75d5b0\"},{\"content\":{\"connectorIds\":[\"RConn1\"],\"side\":\"BOTTOM\"},\"type\":\"ConnectorPlacement.EquallySpacedRectSide\",\"uuid\":\"2353ed68-b1a1-4775-9ca9-31e268d5443b\"}]},\"type\":\"ConnectorPlacement.EquallySpacedConnector\",\"uuid\":\"d5479f4c-4e65-4791-adcb-73df11f88590\"}],\"packageUris\":[\"http://schema.mathworks.com/mf0/Connector/R2020b\"],\"version\":\"1.0\"}"
  D : PMIOPort  Side=Left
  S : PMIOPort  Port=2  Side=Left
  m : Outport
  wires:
  Bus Creator/1 -> m/1
  [mosfet_HA_temp_Q1] -> Bus Creator/5  "mosfet_HA_temp_Q1"
  [mosfet_JH_temp_Q1] -> Bus Creator/4  "mosfet_JH_temp_Q1"
  [mosfet_current_Q1] -> Bus Creator/3  "mosfet_current_Q1"
  [mosfet_voltage_Q1] -> Bus Creator/2  "mosfet_voltage_Q1"
  [mosfet_ploss_Q1] -> Bus Creator/1  "mosfet_ploss_Q1"
  G/1 -> Simulink-PS Converter/1
  [ic_zvs_Q1] -> Bus Creator/6  "ic_zvs_Q1"
  connections:
  mosfet_thermal_1/LConn1 -- Simulink-PS Converter/RConn1
  mosfet_thermal_1/LConn2 -- D/RConn1
  S/RConn1 -- mosfet_thermal_1/RConn1

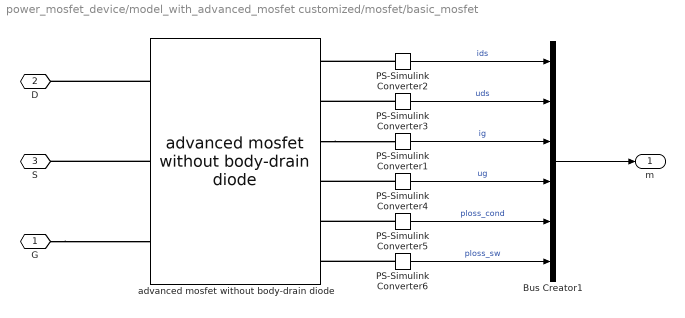
== system power_mosfet_device/model_with_advanced_mosfet customized/mosfet/basic_mosfet ==
  Bus Creator1 : BusCreator  Inputs=6
  PS-Simulink Converter1 : nesl_utility/PS-Simulink Converter  PhysicalDomain=network_engine_domain  SubClassName=ps_output  LeftPortType=input  RightPortType=output  PseudoPeriodic=off  Frequencies=[]  VectorFormat=1-D array  Unit=A  AffineConversion=off
  PS-Simulink Converter2 : nesl_utility/PS-Simulink Converter  PhysicalDomain=network_engine_domain  SubClassName=ps_output  LeftPortType=input  RightPortType=output  PseudoPeriodic=off  Frequencies=[]  VectorFormat=1-D array  Unit=A  AffineConversion=off
  PS-Simulink Converter3 : nesl_utility/PS-Simulink Converter  PhysicalDomain=network_engine_domain  SubClassName=ps_output  LeftPortType=input  RightPortType=output  PseudoPeriodic=off  Frequencies=[]  VectorFormat=1-D array  Unit=V  AffineConversion=off
  PS-Simulink Converter4 : nesl_utility/PS-Simulink Converter  PhysicalDomain=network_engine_domain  SubClassName=ps_output  LeftPortType=input  RightPortType=output  PseudoPeriodic=off  Frequencies=[]  VectorFormat=1-D array  Unit=V  AffineConversion=off
  PS-Simulink Converter5 : nesl_utility/PS-Simulink Converter  PhysicalDomain=network_engine_domain  SubClassName=ps_output  LeftPortType=input  RightPortType=output  PseudoPeriodic=off  Frequencies=[]  VectorFormat=1-D array  Unit=W  AffineConversion=off
  PS-Simulink Converter6 : nesl_utility/PS-Simulink Converter  PhysicalDomain=network_engine_domain  SubClassName=ps_output  LeftPortType=input  RightPortType=output  PseudoPeriodic=off  Frequencies=[]  VectorFormat=1-D array  Unit=W  AffineConversion=off
  advanced mosfet without body-drain diode : advanced_mosfet_lib/advanced mosfet without body-drain diode  Vth=Vth_m V  g_fs=g_fs_m A/V  Rds_on=Rds_on_m Ohm  Cgs=Cgs_m F  Cgd=Cgd_m F  Cds=Cds_m F  Rg=Rgate_internal_m Ohm  Eon=Eon_m J  Eoff=Eoff_m J  Err=Err_m J  Voff_sw_loss=Voff_sw_loss_m V  Ion_sw_loss=Ion_sw_loss_m A  ids_i_specify=off  ids_i_priority=None  ids_i=0 A  ids_i_nominal_specify=off  ids_i_nominal_value=1  ids_i_nominal_unit=A  ids_ii_specify=off  ids_ii_priority=None  ids_ii=0 A  ids_ii_nominal_specify=off  ids_ii_nominal_value=1  ids_ii_nominal_unit=A  idsi_specify=off  idsi_priority=High  idsi=0 A  idsi_nominal_specify=off  idsi_nominal_value=1  idsi_nominal_unit=A  icgs_specify=off  icgs_priority=None  icgs=0 A  icgs_nominal_specify=off  icgs_nominal_value=1  icgs_nominal_unit=A  icgd_specify=off  icgd_priority=None  icgd=0 A  icgd_nominal_specify=off  icgd_nominal_value=1  icgd_nominal_unit=A  icds_specify=off  icds_priority=None  icds=0 A  icds_nominal_specify=off  icds_nominal_value=1  icds_nominal_unit=A  ugs_specify=off  ugs_priority=None  ugs=0 V  ugs_nominal_specify=off  ugs_nominal_value=1  ugs_nominal_unit=V  uds_specify=off  uds_priority=None  uds=0 V  uds_nominal_specify=off  uds_nominal_value=1  uds_nominal_unit=V  ucgs_specify=off  ucgs_priority=None  ucgs=0 V  ucgs_nominal_specify=off  ucgs_nominal_value=1  ucgs_nominal_unit=V  ucgd_specify=off  ucgd_priority=None  ucgd=0 V  ucgd_nominal_specify=off  ucgd_nominal_value=1  ucgd_nominal_unit=V  udsi_specify=off  udsi_priority=None  udsi=0 V  udsi_nominal_specify=off  udsi_nominal_value=1  udsi_nominal_unit=V  igs_specify=off  igs_priority=High  igs=0 A  igs_nominal_specify=off  igs_nominal_value=1  igs_nominal_unit=A  idsi_active_specify=off  idsi_active_priority=None  idsi_active=0 A  idsi_active_nominal_specify=off  idsi_active_nominal_value=1  idsi_active_nominal_unit=A  idsi_on_specify=off  idsi_on_priority=None  idsi_on=0 A  idsi_on_nominal_specify=off  idsi_on_nominal_value=1  idsi_on_nominal_unit=A
      settings: InternalSimscapePortConfiguration="{\"Bottom\":[],\"Left\":[{\"id\":\"D\",\"label\":\"D\",\"type\":\"foundation.electrical.electrical\"},{\"id\":\"S\",\"label\":\"S\",\"type\":\"foundation.electrical.electrical\"},{\"id\":\"G\",\"label\":\"G\",\"type\":\"foundation.electrical.electrical\"}],\"Right\":[{\"id\":\"idsi_out\",\"label\":\"ids\",\"type\":\"output\"},{\"id\":\"udsi_out\",\"label\":\"uds\",\"type\":\"output\"},{\"id\":\"igs_out\",\"label\":\"igs\",\"type\":\"output\"},{\"id\":\"ugs_out\",\"label\":\"ugs\",\"type\":\"output\"},{\"id\":\"ploss_cond\",\"label\":\"ploss_cond\",\"type\":\"output\"},{\"id\":\"ploss_sw\",\"label\":\"ploss_sw\",\"type\":\"output\"}],\"Top\":[]}"
  G : PMIOPort  Side=Left
  D : PMIOPort  Port=2  Side=Left
  S : PMIOPort  Port=3  Side=Right
  m : Outport
  wires:
  Bus Creator1/1 -> m/1
  PS-Simulink Converter2/1 -> Bus Creator1/1  "ids"
  PS-Simulink Converter3/1 -> Bus Creator1/2  "uds"
  PS-Simulink Converter1/1 -> Bus Creator1/3  "ig"
  PS-Simulink Converter4/1 -> Bus Creator1/4  "ug"
  PS-Simulink Converter5/1 -> Bus Creator1/5  "ploss_cond"
  PS-Simulink Converter6/1 -> Bus Creator1/6  "ploss_sw"
  connections:
  PS-Simulink Converter3/LConn1 -- advanced mosfet without body-drain diode/RConn2
  PS-Simulink Converter2/LConn1 -- advanced mosfet without body-drain diode/RConn1
  advanced mosfet without body-drain diode/LConn1 -- D/RConn1
  advanced mosfet without body-drain diode/LConn2 -- S/RConn1
  G/RConn1 -- advanced mosfet without body-drain diode/LConn3
  PS-Simulink Converter4/LConn1 -- advanced mosfet without body-drain diode/RConn4
  advanced mosfet without body-drain diode/RConn3 -- PS-Simulink Converter1/LConn1
  PS-Simulink Converter5/LConn1 -- advanced mosfet without body-drain diode/RConn5
  PS-Simulink Converter6/LConn1 -- advanced mosfet without body-drain diode/RConn6
